simulink model "plant_model"  (R2023b)
settings: Solver=VariableStepAuto  StartTime=0.0  StopTime=10.0  RelTol=1e-3
undefined symbols (not defined in the file): param, sysc, x0
libraries: nesl_utility x4, fl_lib x3, SimscapeFluids_lib x2
settings Model: Creator=MPC5  LastModifiedBy=MPC5

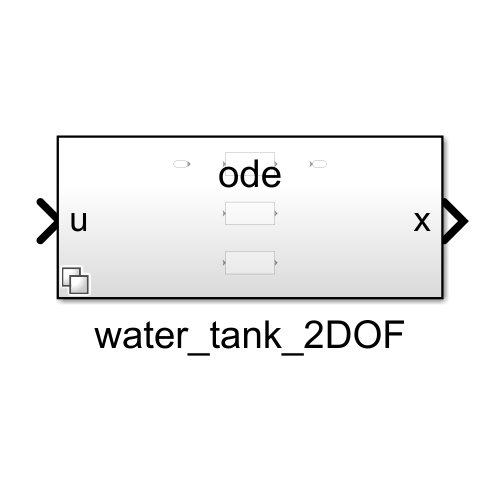
[thumbnail: Simulink's stored preview of the top-level diagram]
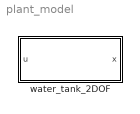
== system plant_model ==
  water_tank_2DOF : Subsystem  Variant=on

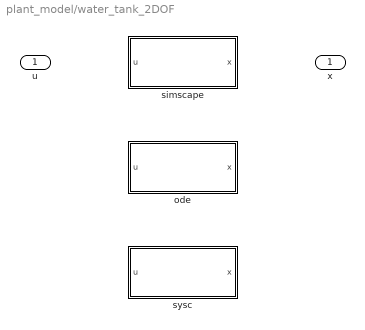
== system plant_model/water_tank_2DOF ==
  u : Inport
  ode : Subsystem  VariantControl="plant_model_type==\"ode\""
  simscape : Subsystem  VariantControl="plant_model_type==\"simscape\""
  sysc : Subsystem  VariantControl="plant_model_type==\"sysc\""
  x : Outport

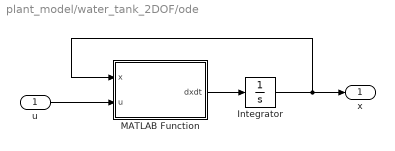
== system plant_model/water_tank_2DOF/ode ==
  u : Inport
  Integrator : Integrator  InitialCondition=x0
  MATLAB Function : MATLAB Function  TreatAsAtomicUnit=on
  x : Outport
  wires:
  MATLAB Function/1(dxdt) -> Integrator/1
  u/1 -> MATLAB Function/2(u)
  Integrator/1 -> x/1, MATLAB Function/1(x)

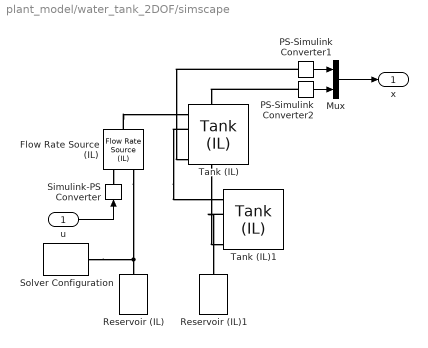
== system plant_model/water_tank_2DOF/simscape ==
  u : Inport
  Flow Rate Source (IL) : fl_lib/Isothermal Liquid/Sources/Flow Rate Source (IL)  source_type=foundation.enum.constant_controlled.controlled  flow_type=foundation.enum.mass_volumetric_flow.volumetric  mass_flow=0 kg/s  volumetric_flow=0 m^3/s
      settings: InternalSimscapePortConfiguration="{\"Bottom\":[],\"Left\":[{\"id\":\"A\",\"label\":\"A\",\"type\":\"foundation.isothermal_liquid.isothermal_liquid\"},{\"id\":\"V\",\"label\":\"V\",\"type\":\"input\"}],\"Right\":[{\"id\":\"B\",\"label\":\"B\",\"type\":\"foundation.isothermal_liquid.isothermal_liquid\"}],\"Top\":[]}"
  Mux : Mux  Inputs=2
  PS-Simulink Converter1 : nesl_utility/PS-Simulink Converter  PhysicalDomain=network_engine_domain  SubClassName=ps_output  LeftPortType=input  RightPortType=output  PseudoPeriodic=off  Frequencies=[]  VectorFormat=inherit  Unit=inherit  AffineConversion=off
  PS-Simulink Converter2 : nesl_utility/PS-Simulink Converter  PhysicalDomain=network_engine_domain  SubClassName=ps_output  LeftPortType=input  RightPortType=output  PseudoPeriodic=off  Frequencies=[]  VectorFormat=inherit  Unit=inherit  AffineConversion=off
  Reservoir (IL) : fl_lib/Isothermal Liquid/Elements/Reservoir (IL)  reservoir_type=foundation.enum.constant_controlled.constant  pressure_spec=foundation.enum.pressure_spec.atmospheric  reservoir_pressure=0.101325 MPa
  Reservoir (IL)1 : fl_lib/Isothermal Liquid/Elements/Reservoir (IL)  reservoir_type=foundation.enum.constant_controlled.constant  pressure_spec=foundation.enum.pressure_spec.atmospheric  reservoir_pressure=0.101325 MPa
  Simulink-PS Converter : nesl_utility/Simulink-PS Converter  PhysicalDomain=network_engine_domain  SubClassName=ps_input  LeftPortType=input  RightPortType=output  PseudoPeriodic=off  Frequencies=[]  NoiseDistribution=none  NoiseParameters=[]  Unit=1  AffineConversion=off  FilteringAndDerivatives=provide  SimscapeFilterOrder=1  InputFilterTimeConstant=0.001  UdotUserProvided=0
  Solver Configuration : nesl_utility/Solver Configuration  PhysicalDomain=network_engine_domain  SubClassName=solver  LeftPortType=input  RightPortType=generic  Tones=[]  Harmonics=[]  SimulateNoise=off  Profile=off  UseLocalSampling=off  EnableSwitchedLinearOptims=on  FrequencyDomain=off  UseCCode=off  RelTol=0.001  AbsTol=0.001  MinStep=1e-09  ToWorkspace=off  RevertToSquareIcSolve=off  NumHomotopyIterations=100  PhasorMode=off  PhasorModeNumHarmonics=1  ConsistencySolver=NEWTON_XTOL_AFTER_FTOL  IndexReductionMethod=DerivativeReplacement  DoDC=off  ResidualTolerance=1e-09  ConsistencyTolSource=GLOBAL  ConsistencyAbsTol=0.001  ConsistencyRelTol=0.001  ConsistencyTolFactor=0.001  UseLocalSolver=off  LocalSolverChoice=NE_BACKWARD_EULER_ADVANCER  ResolveIndetEquations=on  FunctionEvalNumThread=1  LocalSolverSampleTime=0.001  DoFixedCost=off  MaxNonlinIter=3  MaxModeIter=2  ComputeImpulses=off  ImpulseIterations=2  LinearAlgebra=auto  LinearAlgebraNumThread=0  EquationFormulation=NE_TIME_EF  DelaysMemoryBudget=1024  AutomaticFiltering=on  FilteringTimeConstant=0.001  PartitionStorageMethod=AS_NEEDED  PartitionMemoryBudget=1024  PartitionMethod=ROBUST  MultibodyUseLocalSolver=off  MultibodyLocalSolverChoice=ODE1  MultibodyLocalSolverSampleTime=0.001
  Tank (IL) : SimscapeFluids_lib/Isothermal Liquid/Tanks & Accumulators/Tank (IL)  num_inlet=fluids.isothermal_liquid.tanks_accumulators.enum.NumInlet.Two  pressure_spec=fluids.isothermal_liquid.tanks_accumulators.enum.TankPressureSpec.Atmospheric  tank_pressure=0.101325 MPa  volume_spec=fluids.isothermal_liquid.tanks_accumulators.enum.TankVolumeSpec.Constant  tank_area=param.A1 m^2  level_TLU=[0, 3, 5] m  volume_TLU=[0, 4, 6] m^3  inlet_height_A=0.1 m  inlet_area_A=0.01 m^2  inlet_height_AB=[inf,0] m  inlet_area_AB=[1,param.a1] m^2  inlet_height_ABC=[.1, .1, .1] m  inlet_area_ABC=[.01, .01, .01] m^2  inlet_height_ABCD=0.1 * ones(1, 4) m  inlet_area_ABCD=0.01 * ones(1, 4) m^2  inlet_height_ABCDE=0.1 * ones(1, 5) m  inlet_area_ABCDE=0.01 * ones(1, 5) m^2  inlet_height_ABCDEF=0.1 * ones(1, 6) m  inlet_area_ABCDEF=0.01 * ones(1, 6) m^2  level_check=simscape.enum.assert.action.none  capacity_check=simscape.enum.assert.action.none  max_capacity=10 m^3  g=param.g m/s^2  level_specify=on  level_priority=High  level=x0(1) m  level_nominal_specify=off  level_nominal_unit=m  level_nominal_value=1  volume_specify=off  volume_priority=None  volume=5 m^3  volume_nominal_specify=off  volume_nominal_unit=m^3  volume_nominal_value=1  mass_specify=off  mass_priority=None  mass=5000 kg  mass_nominal_specify=off  mass_nominal_unit=kg  mass_nominal_value=1
      settings: InternalSimscapePortConfiguration="{\"Bottom\":[],\"Left\":[{\"id\":\"A\",\"label\":\"A\",\"type\":\"foundation.isothermal_liquid.isothermal_liquid\"},{\"id\":\"B\",\"label\":\"B\",\"type\":\"foundation.isothermal_liquid.isothermal_liquid\"}],\"Right\":[],\"Top\":[{\"id\":\"V\",\"label\":\"V\",\"type\":\"output\"},{\"id\":\"L\",\"label\":\"L\",\"type\":\"output\"}]}"
  Tank (IL)1 : SimscapeFluids_lib/Isothermal Liquid/Tanks & Accumulators/Tank (IL)  num_inlet=fluids.isothermal_liquid.tanks_accumulators.enum.NumInlet.Two  pressure_spec=fluids.isothermal_liquid.tanks_accumulators.enum.TankPressureSpec.Atmospheric  tank_pressure=0.101325 MPa  volume_spec=fluids.isothermal_liquid.tanks_accumulators.enum.TankVolumeSpec.Constant  tank_area=param.A2 m^2  level_TLU=[0, 3, 5] m  volume_TLU=[0, 4, 6] m^3  inlet_height_A=0.1 m  inlet_area_A=0.01 m^2  inlet_height_AB=[inf,0] m  inlet_area_AB=[1,param.a2] m^2  inlet_height_ABC=[.1, .1, .1] m  inlet_area_ABC=[.01, .01, .01] m^2  inlet_height_ABCD=0.1 * ones(1, 4) m  inlet_area_ABCD=0.01 * ones(1, 4) m^2  inlet_height_ABCDE=0.1 * ones(1, 5) m  inlet_area_ABCDE=0.01 * ones(1, 5) m^2  inlet_height_ABCDEF=0.1 * ones(1, 6) m  inlet_area_ABCDEF=0.01 * ones(1, 6) m^2  level_check=simscape.enum.assert.action.none  capacity_check=simscape.enum.assert.action.none  max_capacity=10 m^3  g=param.g m/s^2  level_specify=on  level_priority=High  level=x0(2) m  level_nominal_specify=off  level_nominal_unit=m  level_nominal_value=1  volume_specify=off  volume_priority=None  volume=5 m^3  volume_nominal_specify=off  volume_nominal_unit=m^3  volume_nominal_value=1  mass_specify=off  mass_priority=None  mass=5000 kg  mass_nominal_specify=off  mass_nominal_unit=kg  mass_nominal_value=1
      settings: InternalSimscapePortConfiguration="{\"Bottom\":[],\"Left\":[{\"id\":\"A\",\"label\":\"A\",\"type\":\"foundation.isothermal_liquid.isothermal_liquid\"},{\"id\":\"B\",\"label\":\"B\",\"type\":\"foundation.isothermal_liquid.isothermal_liquid\"}],\"Right\":[],\"Top\":[{\"id\":\"V\",\"label\":\"V\",\"type\":\"output\"},{\"id\":\"L\",\"label\":\"L\",\"type\":\"output\"}]}"
  x : Outport
  wires:
  Mux/1 -> x/1
  PS-Simulink Converter2/1 -> Mux/2
  PS-Simulink Converter1/1 -> Mux/1
  u/1 -> Simulink-PS Converter/1
  connections:
  Reservoir (IL)/LConn1 -- Flow Rate Source (IL)/LConn1 -- Solver Configuration/RConn1
  Tank (IL)/LConn2 -- Tank (IL)1/LConn1
  Flow Rate Source (IL)/RConn1 -- Tank (IL)/LConn1
  Flow Rate Source (IL)/LConn2 -- Simulink-PS Converter/RConn1
  PS-Simulink Converter1/LConn1 -- Tank (IL)/LConn4
  PS-Simulink Converter2/LConn1 -- Tank (IL)1/LConn4
  Tank (IL)1/LConn2 -- Reservoir (IL)1/LConn1

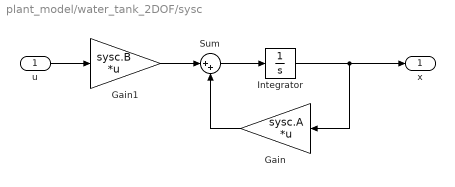
== system plant_model/water_tank_2DOF/sysc ==
  u : Inport
  Gain : Gain  Gain=sysc.A  Multiplication=Matrix(K*u)
  Gain1 : Gain  Gain=sysc.B  Multiplication=Matrix(K*u)
  Integrator : Integrator  InitialCondition=x0
  Sum : Sum  Inputs=|++
  x : Outport
  wires:
  Sum/1 -> Integrator/1
  u/1 -> Gain1/1
  Gain1/1 -> Sum/1
  Gain/1 -> Sum/2
  Integrator/1 -> x/1, Gain/1

== matlab function plant_model/water_tank_2DOF/ode/MATLAB Function ==
  data: x input size=param.xdim; u input size=param.udim; dxdt output size=param.xdim; param parameter
function dxdt = ode(x,u,param)
    dxdt = plant_ode(0,x,u,param);
end
